simulink subsystem "Pendulum"  (R2020b)
settings: Solver=VariableStepAuto  StartTime=0.0  StopTime=10.0  RelTol=1e-3
settings Model: Creator=avina  LastModifiedBy=avina

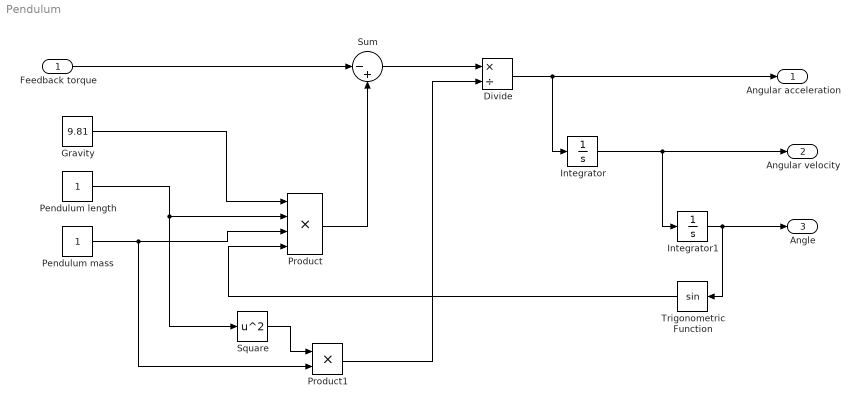
== system Pendulum ==
  Feedback torque : Inport
  Divide : Product  Inputs=*/
  Gravity : Constant  Value=9.81
  Integrator : Integrator
  Integrator1 : Integrator
  Pendulum length : Constant
  Pendulum mass : Constant
  Product : Product  Inputs=4
  Product1 : Product
  Square : Math  Operator=square  SaturateOnIntegerOverflow=on
  Sum : Sum  Inputs=|-+
  Trigonometric Function : Trigonometry
  Angular acceleration : Outport
  Angular velocity : Outport  Port=2
  Angle : Outport  Port=3
  wires:
  Gravity/1 -> Product/1
  Feedback torque/1 -> Sum/1
  Product/1 -> Sum/2
  Sum/1 -> Divide/1
  Pendulum length/1 -> Product/2, Square/1
  Pendulum mass/1 -> Product/3, Product1/2
  Square/1 -> Product1/1
  Product1/1 -> Divide/2
  Divide/1 -> Integrator/1, Angular acceleration/1
  Integrator/1 -> Integrator1/1, Angular velocity/1
  Integrator1/1 -> Trigonometric Function/1, Angle/1
  Trigonometric Function/1 -> Product/4
